simulink model "MLIiBRD7LVL"  (Simulink 7.9)
settings: Solver=ode45  StartTime=0.0  StopTime=1  RelTol=1e-3
libraries: powerlib x13, simulink x4
settings Model: Creator=DILEEP KUMAR  LastModifiedBy=DILEEP KUMAR

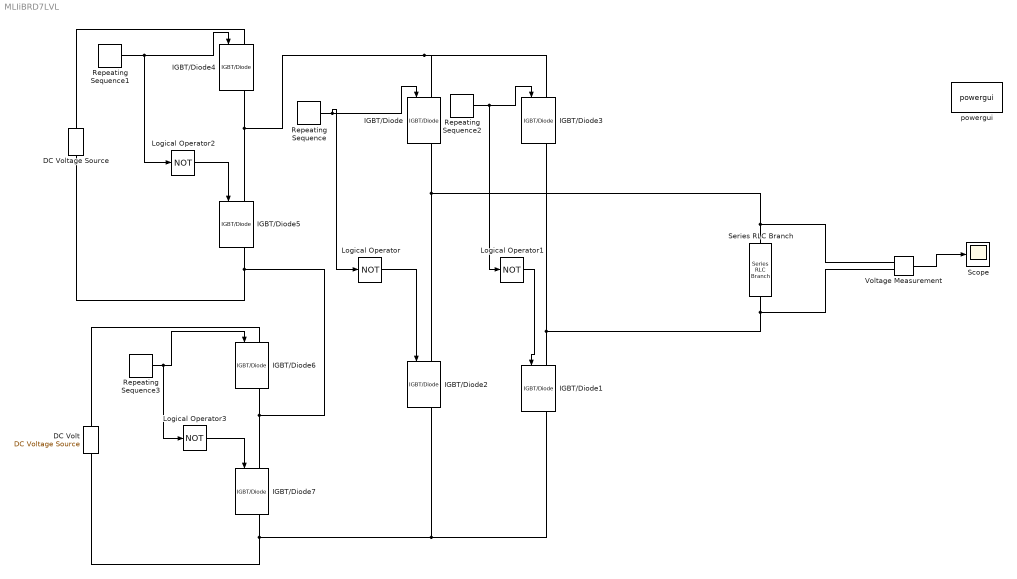
== system MLIiBRD7LVL ==
  DC Volt : powerlib/Electrical Sources/DC Voltage Source  Amplitude=200  Measurements=None
  DC Voltage Source : powerlib/Electrical Sources/DC Voltage Source  Amplitude=100  Measurements=None
  IGBT/Diode{,1..7} (8 alike) : powerlib/Power Electronics/IGBT//Diode  Ron=1e-3  Rs=1e5  Cs=inf  Measurements=on
  Logical Operator{,1..3} (4 alike) : Logic  Operator=NOT  AllPortsSameDT=off  OutDataTypeStr=boolean
  Repeating Sequence : simulink/Sources/Repeating Sequence  rep_seq_t=[0 1 1 7 7 14]*(0.02/14)  rep_seq_y=[0 0 1 1 0 0 ]
  Repeating Sequence1 : simulink/Sources/Repeating Sequence  rep_seq_t=[0 1 1 2 2 3 3 5 5 6 6 7 7 8 8 9 9 10 10 12 12 13 13 14 14]*(0.02/14)  rep_seq_y=[0 0 1 1 0 0 1 1 0 0 1 1 0 0 1 1 0 0 1 1 0 0 1 1 0 ]
  Repeating Sequence2 : simulink/Sources/Repeating Sequence  rep_seq_t=[0 8 8 14 14]*(0.02/14)  rep_seq_y="[0 0 1 1 0  ]"
  Repeating Sequence3 : simulink/Sources/Repeating Sequence  rep_seq_t=[0 2 2 6 6 9 9 13 13 14]*(0.02/14)  rep_seq_y=[0 0 1 1 0 0 1 1 0 0 ]
  Scope : Scope
      settings: SaveName=Ibridge
  Series RLC Branch : powerlib/Elements/Series RLC Branch  LConnTagsString=__new0  RConnTagsString=__new0  BranchType=R  Resistance=10  Inductance=1e-3  SetiL0=off  InitialCurrent=0  Capacitance=1e-6  Setx0=off  InitialVoltage=0  Measurements=None
  Voltage Measurement : powerlib/Measurements/Voltage Measurement  PhasorSimulation=off  OutputType=Complex  PSBequivalent=0
  powergui : powerlib/powergui  Priority=1  SimulationMode=Discrete  SolverType=Tustin  SampleTime=50e-6  frequency=60  SPID=off  DisableSnubberDevices=off  DisableRonSwitches=off  DisableVfSwitches=off  SwTol=0  Interpol=off  DisplayEquations=off  FunctionMessages=off  frequencyindice=0  Pbase=100e6  ErrMax=1e-4  Iterations=50  UnitsV=kV  UnitsW=MW  echomessages=off  HookPort=off  EnableUseOfTLC=off  x0status=blocks  RestoreLinks=warning  ResistiveCurrentMeasurement=off  Ylog=off  Xlog=on  ShowGrid=off  save=off  variable=ZData  structure=Ibridge  ZoomFFT=off  StartTime=0.2  cycles=1  DisplayStyle=1  fundamental=50  FreqAxis=off  MaxFrequency=1000  frequencyindicesteady=1  display=off  methode=off
  wires:
  Repeating Sequence/1 -> IGBT/Diode/1, Logical Operator/1
  Repeating Sequence2/1 -> IGBT/Diode3/1, Logical Operator1/1
  Logical Operator/1 -> IGBT/Diode2/1
  Logical Operator1/1 -> IGBT/Diode1/1
  Repeating Sequence3/1 -> IGBT/Diode6/1, Logical Operator3/1
  Repeating Sequence1/1 -> IGBT/Diode4/1, Logical Operator2/1
  Logical Operator2/1 -> IGBT/Diode5/1
  Logical Operator3/1 -> IGBT/Diode7/1
  Voltage Measurement/1 -> Scope/1
  connections:
  IGBT/Diode2/LConn1 -- IGBT/Diode/RConn1 -- Series RLC Branch/LConn1 -- Voltage Measurement/LConn1
  Series RLC Branch/RConn1 -- IGBT/Diode1/LConn1 -- IGBT/Diode3/RConn1 -- Voltage Measurement/LConn2
  IGBT/Diode5/LConn1 -- IGBT/Diode4/RConn1 -- IGBT/Diode3/LConn1 -- IGBT/Diode/LConn1
  DC Voltage Source/RConn1 -- IGBT/Diode4/LConn1
  IGBT/Diode7/LConn1 -- IGBT/Diode6/RConn1 -- DC Voltage Source/LConn1 -- IGBT/Diode5/RConn1
  DC Volt/RConn1 -- IGBT/Diode6/LConn1
  DC Volt/LConn1 -- IGBT/Diode7/RConn1 -- IGBT/Diode1/RConn1 -- IGBT/Diode2/RConn1
